simulink model "nomotosecondorder"  (R2017b)
settings: Solver=VariableStepAuto  StartTime=0.0  StopTime=10.0  RelTol=1e-3
values from neighbouring files (symbols this model uses):
  tsamp = 10    [run18.m]    (also in run18_plot.m)
  x = lsqcurvefit(F,x0, tdata, rdata)    [run_task_1_2.m]
undefined symbols (not defined in the file or in its folder): delta_c
settings Model: Creator=henningward  LastModifiedBy=henningward

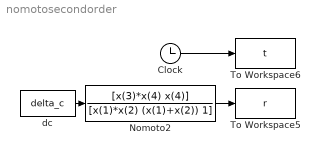
== system nomotosecondorder ==
  Clock : Clock
  Nomoto2 : TransferFcn  Numerator=[x(3)*x(4) x(4)]  Denominator=[x(1)*x(2) (x(1)+x(2)) 1]
  To Workspace5 : ToWorkspace  VariableName=r  SampleTime=tsamp
  To Workspace6 : ToWorkspace  VariableName=t  SampleTime=tsamp
  dc : Constant  Value=delta_c
  wires:
  Nomoto2/1 -> To Workspace5/1
  Clock/1 -> To Workspace6/1
  dc/1 -> Nomoto2/1
